simulink model "si_verification"  (R2021b)
settings: Solver=ode4  StartTime=0.0  StopTime=458  FixedStep=.002  RelTol=1e-3
values from neighbouring files (symbols this model uses):
  k = 1    [Inverted_Pendulum.m]    (also in si_elbow.m = k - gamma*dJdk)
  wc = 10*pi    (= 31.4159265359)    [si_elbow.m]
libraries: cstblocks x3
settings Model: Creator=johnc  LastModifiedBy=johnc

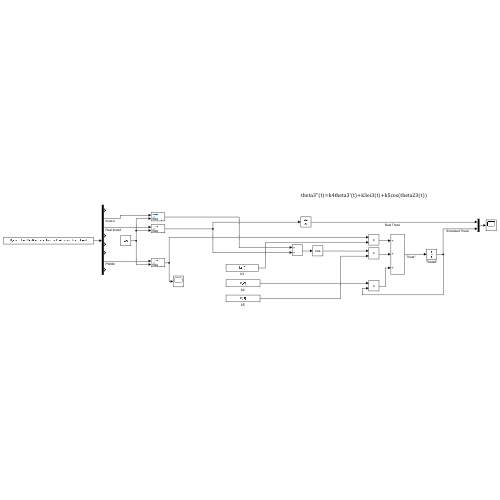
[thumbnail: Simulink's stored preview of the top-level diagram]
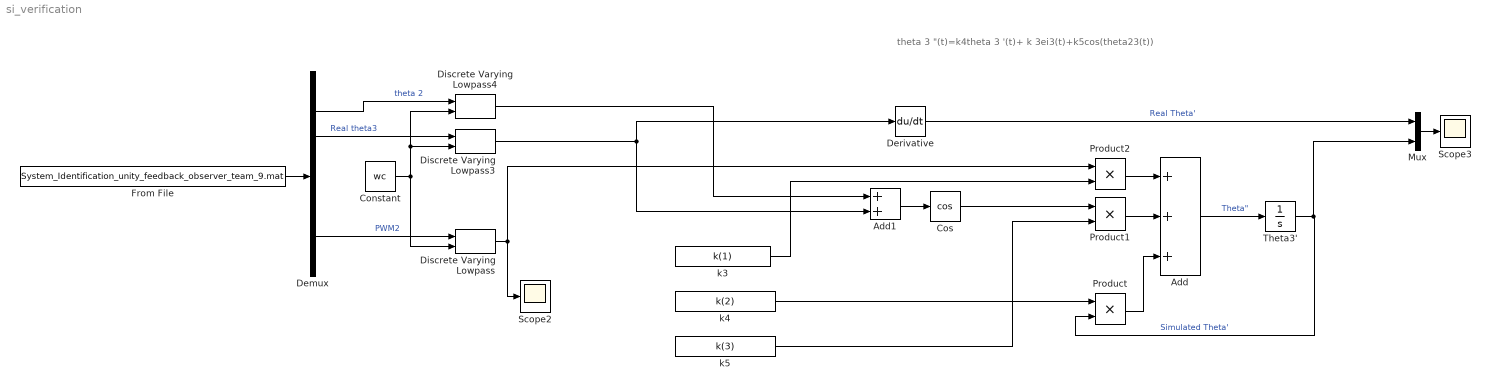
== system si_verification ==
  note: theta 3 "(t)=k4theta 3 '(t)+ k 3ei3(t)+k5cos(theta23(t))
  Add : Sum  Inputs=+++
  Add1 : Sum
  Constant : Constant  Value=wc
  Cos : Trigonometry  Operator=cos
  Demux : Demux  Outputs=8
  Derivative : Derivative
  Discrete Varying Lowpass : cstblocks/Linear Parameter Varying/Discrete Varying Lowpass  N=2  w0=0  Ts=.002
      settings: SourceProductBaseCode=CT
  Discrete Varying Lowpass3 : cstblocks/Linear Parameter Varying/Discrete Varying Lowpass  N=2  w0=0  Ts=.002
      settings: SourceProductBaseCode=CT
  Discrete Varying Lowpass4 : cstblocks/Linear Parameter Varying/Discrete Varying Lowpass  N=2  w0=0  Ts=.002
      settings: SourceProductBaseCode=CT
  From File : FromFile  FileName=System_Identification_unity_feedback_observer_team_9.mat  SampleTime=0
  Mux : Mux  Inputs=2
  Product : Product
  Product1 : Product
  Product2 : Product
  Scope2 : Scope
  Scope3 : Scope
  Theta3' : Integrator
  k3 : Constant  Value=k(1)
  k4 : Constant  Value=k(2)
  k5 : Constant  Value=k(3)
  wires:
  From File/1 -> Demux/1
  Theta3'/1 -> Mux/2, Product/2  "Simulated Theta'"
  Add/1 -> Theta3'/1  "Theta\""
  Product/1 -> Add/3
  Cos/1 -> Product1/1
  Add1/1 -> Cos/1
  Product1/1 -> Add/2
  Product2/1 -> Add/1
  k3/1 -> Product2/2
  k4/1 -> Product/1
  k5/1 -> Product1/2
  Demux/2 -> Discrete Varying Lowpass4/1  "theta 2"
  Demux/3 -> Discrete Varying Lowpass3/1  "Real theta3"
  Demux/7 -> Discrete Varying Lowpass/1  "PWM2"
  Discrete Varying Lowpass3/1 -> Derivative/1, Add1/2
  Discrete Varying Lowpass/1 -> Scope2/1, Product2/1
  Discrete Varying Lowpass4/1 -> Add1/1
  Constant/1 -> Discrete Varying Lowpass4/2, Discrete Varying Lowpass3/2, Discrete Varying Lowpass/2
  Mux/1 -> Scope3/1
  Derivative/1 -> Mux/1  "Real Theta'"
